simulink model "chap02_128"  (R2020a)
settings: Solver=VariableStepAuto  StartTime=0.0  StopTime=10.0  RelTol=1e-3
settings Model: DataTypeOverride=Double  MinMaxOverflowLogging=ForceOff  Creator=chen_w3  LastModifiedBy=chen_w3

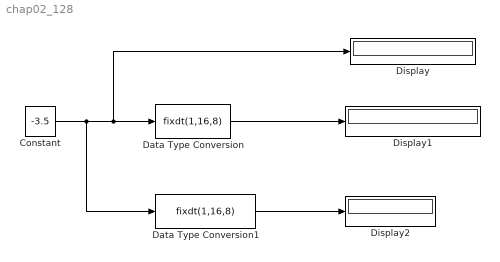
== system chap02_128 ==
  Constant : Constant  Value=-3.5  OutDataTypeStr=fixdt(1,8,3, 'DataTypeOverride', 'Off')  SampleTime=-1
      settings: AttributesFormatString=%<OutDataTypeStr>
  Data Type Conversion : DataTypeConversion  OutDataTypeStr=fixdt(1,16,8)
      settings: AttributesFormatString=|
      | %<ConvertRealWorld>
      | %<OutDataTypeStr>
  Data Type Conversion1 : DataTypeConversion  OutDataTypeStr=fixdt(1,16,8)  ConvertRealWorld=Stored Integer (SI)
      settings: AttributesFormatString=|
      | %<OutDataTypeStr>
      | %<ConvertRealWorld>
  Display : Display
      settings: AttributesFormatString=%<Format>  Format=binary (Stored Integer)
  Display1 : Display
      settings: AttributesFormatString=%<Format>  Format=binary (Stored Integer)
  Display2 : Display
      settings: AttributesFormatString=%<Format>  Format=binary (Stored Integer)
  wires:
  Constant/1 -> Data Type Conversion1/1, Display/1, Data Type Conversion/1
  Data Type Conversion/1 -> Display1/1
  Data Type Conversion1/1 -> Display2/1
